simulink model "h2omnix"  (R2023a)
settings: Solver=ode4  StartTime=0.0  StopTime=inf  RelTol=1e-3
undefined symbols (not defined in the file or in its folder): K_av, Kd_pose, Ki_vel, Kp_pose, Kp_vel
libraries: ros2lib x4, MarineRoboticsLib_2 x3, robotcorelib x1
settings Model: Creator=dnad  LastModifiedBy=Enio
settings OptimizationCC: ReuseModelBlockBuffer=off

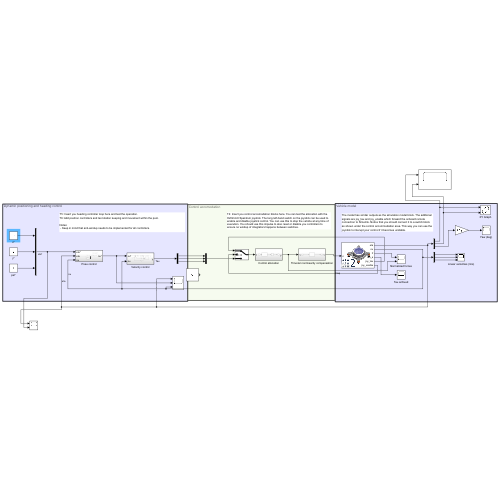
[thumbnail: Simulink's stored preview of the top-level diagram]
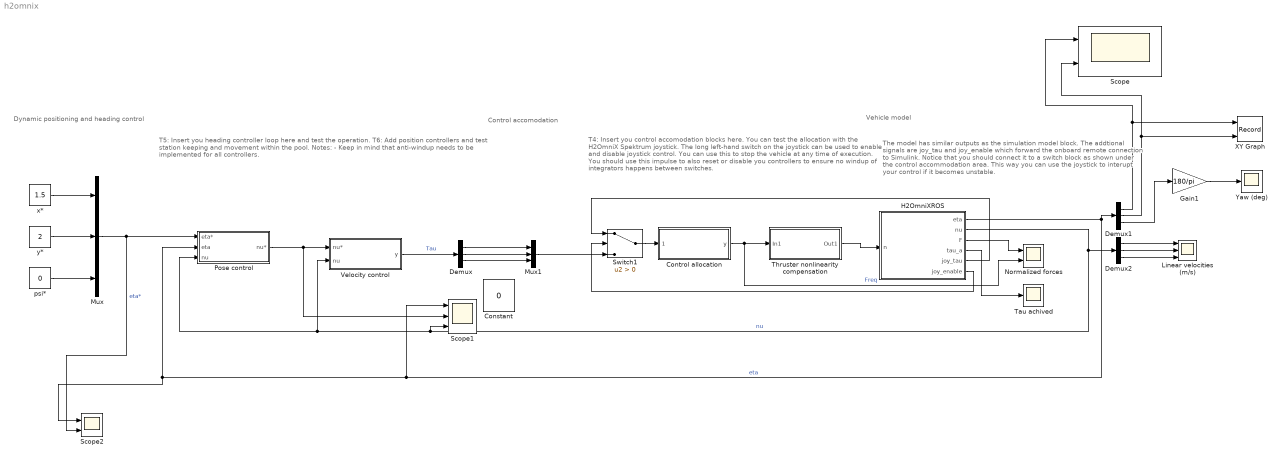
== system h2omnix ==
  note: Control accomodation
  note: T4: Insert you control accomodation blocks here. You can test the allocation with the
      | H2OmniX Spektrum joystick. The long left-hand switch on the joystick can be used to enable and disable joystick control. You can use this to stop the vehicle at any time of execution. You should use this impulse to also reset or disable you controllers to ensure no windup of integrators happens between switches.
  note: Dynamic positioning and heading control
  note: Vehicle model
  note: T5: Insert you heading controller loop here and test the operation.
      | T6: Add position controllers and test station keeping and movement within the pool.
      |
      | Notes:
      |  - Keep in mind that anti-windup needs to be implemented for all controllers.
  note: The model has similar outputs as the simulation model block. The addtional
      | signals are joy_tau and joy_enable which forward the onboard remote
      | connection to Simulink. Notice that you should connect it to a switch block
      | as shown under the control accommodation area. This way you can use the
      | joystick to interupt your control if it becomes unstable.
  Constant : Constant  Value=0
  Control allocation : Subsystem
  Demux : Demux  Outputs=3
  Demux1 : Demux  Outputs=3
  Demux2 : Demux  Outputs=3
  Gain1 : Gain  Gain=180/pi
  H2OmniXROS : Subsystem  AncestorBlock=MarineRoboticsLib_2/H2OmniXROS  mask{vehicle_name=vis, max_pwm=1, pwm_topic=/vis/pwm_out, joy_topic=/vis/joy, odometry_topic=/vis/odometry/filtered}
      mask prompts: vehicle_name "Vehicle name"; max_pwm "Maximum allowed PWM"; pwm_topic "Command"; joy_topic "Joystick"; odometry_topic "Odometry"
      mask init:
      | set_param(gcb, 'pwm_topic',strcat('/', vehicle_name, '/pwm_out'));
      |     set_param(gcb, 'odometry_topic', strcat('/', vehicle_name, '/odometry/filtered'));
      |     set_param(gcb, 'joy_topic', strcat('/', vehicle_name, '/joy'));
      settings: LibrarySourceBlock=MarineRoboticsLib_2/H2OmniXROS
      mask TypeOptions pwm_topic: PublishToROS/topic
      mask TypeOptions joy_topic: Subscribe2/topic
      mask TypeOptions odometry_topic: Subscribe1/topic
      mask DialogControl G1 Prompt: Topics
      mask Display: image('$imagefile'); % Use "Edit Image" on toolstrip to change.
  Linear velocities (m/s) : Scope  NumInputPorts=3
  Mux : Mux  Inputs=3
  Mux1 : Mux  Inputs=3
  Normalized forces : Scope  NumInputPorts=2
  Pose control : Subsystem
  Scope : Scope  NumInputPorts=2
  Scope1 : Scope  NumInputPorts=3
  Scope2 : Scope  NumInputPorts=2
  Switch1 : Switch  Criteria=u2 > Threshold  SaturateOnIntegerOverflow=off  InputSameDT=off
  Tau achived : Scope
  Thruster nonlinearity compensation : Subsystem
  Velocity control : Subsystem
  XY Graph : Record  FileSettingsInternal="{\"entries\":[{\"content\":{\"excelSettings\":{\"content\":{},\"type\":\"Streamout.ExcelSettings\"}},\"type\":\"Streamout.FileSettingStorage\",\"uuid\":\"\"}],\"packageUris\":[\"http:\\/\\/schema.mathworks.com\\/mf0\\/streamout_blocks\\/R2020a\"],\"version\":\"1.0\"}"  Layout=[1 1]  SignalsInternal="{\"entries\":[{\"content\":{\"signals\":[{\"content\":{\"blockPath\":[],\"dimensions\":[1,1],\"domain\":\"\",\"lineColor\":\"#a2142f\",\"plots\":[1],\"port\":1,\"sid\":[\"\"],\"signalID\":29427,\"signalName\":\"Demux1:1\"},\"type\":\"RecordBlkView.Signal\",\"uuid\":\"\"},{\"content\":{\"blockPath\":[],\"dimensions\":[1,1],\"domain\":\"\",\"lineColor\":\"#139fff\",\"plots\":[1],\"port\":2,\"sid\":[\"\"],\"signalID\":29431,\"signalName\":\"Demux1:2\"},\"type\":\"RecordBlkView.Signal\",\"uuid\":\"\"}]},\"type\":\"RecordBlkView.InputSignals\",\"uuid\":\"\"}],\"packageUris\":[\"http:\\/\\/schema.mathworks.com\\/mf0\\/streamout_blocks\\/R2020a\"],\"version\":\"1.0\"}"  VisualizationBindings="{\"xyplotplugin\":{\"info\":[{\"series\":[{\"bindingParametersList\":[{\"parameter\":\"X-Axis\",\"signalID\":29427,\"signalName\":\"Demux1:1\"},{\"parameter\":\"Y-Axis\",\"signalID\":29431,\"signalName\":\"Demux1:2\"}],\"seriesID\":31628}],\"subplotID\":1}]}}"  CompatibilityTag=XY
  Yaw (deg) : Scope
  psi* : Constant  Value=0
  x* : Constant  Value=1.5
  y* : Constant  Value=2
  wires:
  Demux2/1 -> Linear velocities (m/s)/1
  H2OmniXROS/4(tau_a) -> Tau achived/1
  y*/1 -> Mux/2
  Thruster nonlinearity compensation/1(Out1) -> H2OmniXROS/1(n)
  H2OmniXROS/1(eta) -> Scope1/1, Pose control/2(eta), Scope2/1, Demux1/1  "eta"
  Control allocation/1(y) -> Thruster nonlinearity compensation/1(In1), Normalized forces/2  "Freq"
  psi*/1 -> Mux/3
  H2OmniXROS/3(F) -> Normalized forces/1
  Demux1/2 -> XY Graph/2, Scope/2
  H2OmniXROS/2(nu) -> Scope1/3, Pose control/3(nu), Velocity control/2(nu), Demux2/1  "nu"
  Demux1/1 -> XY Graph/1, Scope/1
  Gain1/1 -> Yaw (deg)/1
  Demux1/3 -> Gain1/1
  Demux2/2 -> Linear velocities (m/s)/2
  x*/1 -> Mux/1
  Demux2/3 -> Linear velocities (m/s)/3
  Switch1/1 -> Control allocation/1(1)
  H2OmniXROS/6(joy_enable) -> Switch1/2
  H2OmniXROS/5(joy_tau) -> Switch1/1
  Velocity control/1(y) -> Demux/1  "Tau"
  Mux1/1 -> Switch1/3
  Mux/1 -> Scope2/2, Pose control/1(eta*)  "eta*"
  Pose control/1(nu*) -> Scope1/2, Velocity control/1(nu*)
  Demux/1 -> Mux1/1
  Demux/2 -> Mux1/2
  Demux/3 -> Mux1/3

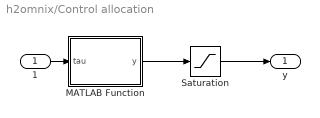
== system h2omnix/Control allocation ==
  1 : Inport
  MATLAB Function : MATLAB Function  TreatAsAtomicUnit=on
  Saturation : Saturate  UpperLimit=1  LowerLimit=-1
  y : Outport
  wires:
  1/1 -> MATLAB Function/1(tau)
  MATLAB Function/1(y) -> Saturation/1
  Saturation/1 -> y/1

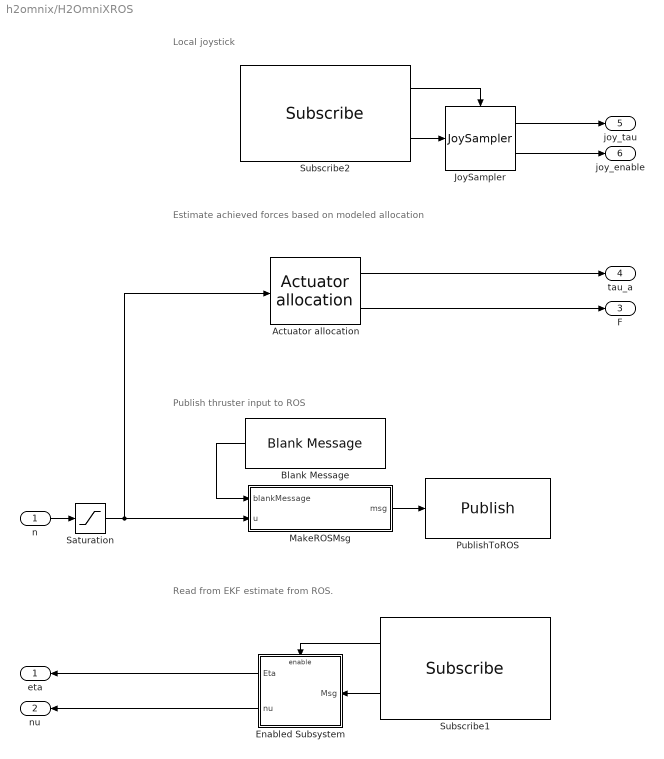
== system h2omnix/H2OmniXROS ==
  note: Local joystick
  note: Read from EKF estimate from ROS.
  note: Publish thruster input to ROS
  note: Estimate achieved forces based on modeled allocation
  n : Inport
  Actuator allocation : MarineRoboticsLib_2/Actuator allocation  Tm=0  B="[0.25, 0.25, -0.25, -0.25; -0.25,  0.25, -0.25,  0.25; -0.25, 0.25, 0.25, -0.25]"  Keff=[1,1,1,1]
  Blank Message : ros2lib/Blank Message  messageClass=Message  entityType=std_msgs/Float32MultiArray  messageType=std_msgs/Float32MultiArray  SampleTime=0.05
  Enabled Subsystem : Subsystem  TreatAsAtomicUnit=on
  JoySampler : MarineRoboticsLib_2/JoyOverROS/JoySampler  SystemSampleTime=-1  VariantActivationTime=update diagram  Latency=0  AutoFrameSizeCalculation=off
  MakeROSMsg : MATLAB Function  TreatAsAtomicUnit=on  SystemSampleTime=0.05
  PublishToROS : ros2lib/Publish  topicSource=Select from ROS network  topic=/vis/pwm_out  messageType=std_msgs/Float32MultiArray  QOSHistory=Keep last  QOSDepth=1  QOSReliability=Reliable  QOSDurability=Volatile
  Saturation : Saturate  UpperLimit=max_pwm  LowerLimit=-max_pwm
  Subscribe1 : ros2lib/Subscribe  topicSource=Specify your own  topic=/vis/odometry/filtered  messageType=nav_msgs/Odometry  sampleTime=0.05  QOSHistory=Keep last  QOSDepth=1  QOSReliability=Reliable  QOSDurability=Volatile
  Subscribe2 : ros2lib/Subscribe  topicSource=Specify your own  topic=/vis/joy  messageType=sensor_msgs/Joy  sampleTime=0.05  QOSHistory=Keep last  QOSDepth=1  QOSReliability=Reliable  QOSDurability=Volatile
  eta : Outport
  nu : Outport  Port=2
  F : Outport  Port=3
  tau_a : Outport  Port=4
  joy_tau : Outport  Port=5
  joy_enable : Outport  Port=6
  wires:
  Saturation/1 -> Actuator allocation/1, MakeROSMsg/2(u)
  MakeROSMsg/1(msg) -> PublishToROS/1
  Subscribe1/2 -> Enabled Subsystem/1(Msg)
  Subscribe1/1 -> Enabled Subsystem/Enable
  Enabled Subsystem/1(Eta) -> eta/1
  Blank Message/1 -> MakeROSMsg/1(blankMessage)
  n/1 -> Saturation/1
  Enabled Subsystem/2(nu) -> nu/1
  Actuator allocation/2 -> F/1
  Actuator allocation/1 -> tau_a/1
  JoySampler/2 -> joy_enable/1
  Subscribe2/2 -> JoySampler/1
  JoySampler/1 -> joy_tau/1
  Subscribe2/1 -> JoySampler/Enable

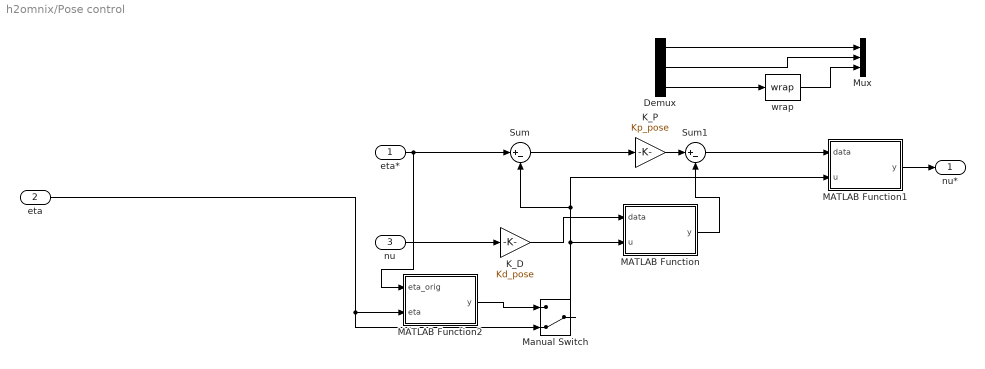
== system h2omnix/Pose control ==
  eta* : Inport
  eta : Inport  Port=2
  nu : Inport  Port=3
  Demux : Demux  Outputs=3
  K_D : Gain  Gain=Kd_pose
  K_P : Gain  Gain=Kp_pose
  MATLAB Function : MATLAB Function  TreatAsAtomicUnit=on
  MATLAB Function1 : MATLAB Function  TreatAsAtomicUnit=on
  MATLAB Function2 : MATLAB Function  TreatAsAtomicUnit=on
  Manual Switch : ManualSwitch  CurrentSetting=0
  Mux : Mux  Inputs=3
  Sum : Sum  Inputs=|+-
  Sum1 : Sum  Inputs=|+-
  wrap : MarineRoboticsLib_2/wrap  SystemSampleTime=-1  VariantActivationTime=update diagram  Latency=0  AutoFrameSizeCalculation=off
      settings: LibrarySourceBlock=|
      | simulink/User-Defined
      | Functions/MATLAB Function
  nu* : Outport
  wires:
  eta*/1 -> MATLAB Function2/1(eta_orig), Sum/1
  nu/1 -> K_D/1
  K_D/1 -> MATLAB Function/1(data)
  MATLAB Function/1(y) -> Sum1/2
  MATLAB Function1/1(y) -> nu*/1
  eta/1 -> Manual Switch/2, MATLAB Function2/2(eta)
  MATLAB Function2/1(y) -> Manual Switch/1
  Manual Switch/1 -> MATLAB Function/2(u), MATLAB Function1/2(u), Sum/2
  Demux/3 -> wrap/1
  wrap/1 -> Mux/3
  Demux/1 -> Mux/1
  Demux/2 -> Mux/2
  Sum1/1 -> MATLAB Function1/1(data)
  K_P/1 -> Sum1/1
  Sum/1 -> K_P/1

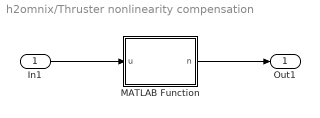
== system h2omnix/Thruster nonlinearity compensation ==
  In1 : Inport
  MATLAB Function : MATLAB Function  TreatAsAtomicUnit=on
  Out1 : Outport
  wires:
  In1/1 -> MATLAB Function/1(u)
  MATLAB Function/1(n) -> Out1/1

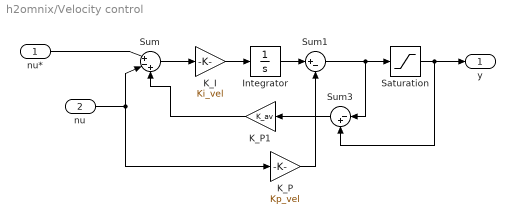
== system h2omnix/Velocity control ==
  nu* : Inport
  nu : Inport  Port=2
  Integrator : Integrator
  K_I : Gain  Gain=Ki_vel
  K_P : Gain  Gain=Kp_vel
  K_P1 : Gain  Gain=K_av
  Saturation : Saturate
  Sum : Sum  Inputs=|+-+
  Sum1 : Sum  Inputs=|+-
  Sum3 : Sum  Inputs=|-+
  y : Outport
  wires:
  nu*/1 -> Sum/1
  nu/1 -> K_P/1, Sum/2
  K_P/1 -> Sum1/2
  Sum1/1 -> Sum3/1, Saturation/1
  Saturation/1 -> y/1, Sum3/2
  Integrator/1 -> Sum1/1
  Sum3/1 -> K_P1/1
  K_I/1 -> Integrator/1
  Sum/1 -> K_I/1
  K_P1/1 -> Sum/3

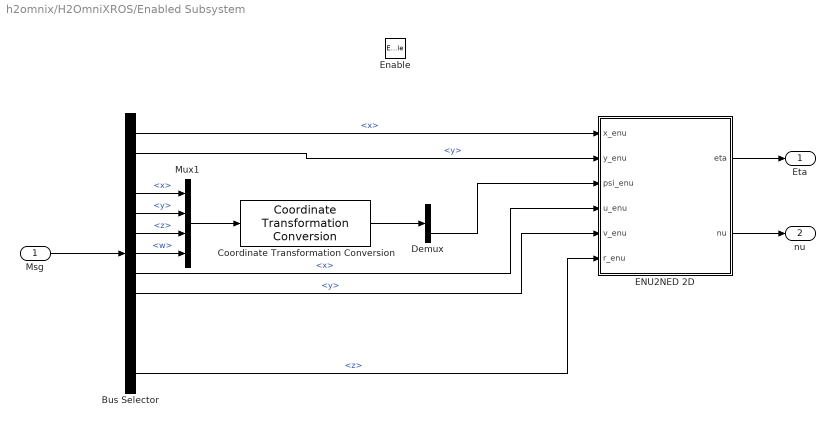
== system h2omnix/H2OmniXROS/Enabled Subsystem ==
  Msg : Inport
  Enable : EnablePort
  Bus Selector : BusSelector  OutputSignals=pose.pose.position.x,pose.pose.position.y,pose.pose.position.z,pose.pose.orientation.x,pose.pose.orientation.y,pose.pose.orientation.z,pose.pose.orientation.w,twist.twist.linear.x,twist.twist.linear.y,twist.twist.linear.z,twist.twist.angular.x,twist.twist.angular.y,twist.twist.angular.z
  Coordinate Transformation Conversion : robotcorelib/Coordinate Transformation Conversion  InputRepresentation=Quaternion  InputEulerSequence=ZYX  ShowTrVecInputPort=on  OutputRepresentation=Euler Angles  OutputEulerSequence=ZYX  ShowTrVecOutputPort=on  SimulateUsing=Interpreted execution
      settings: LibrarySourceBlock=roslib/Utilities/Coordinate Transformation Conversion
  Demux : Demux  Outputs=3
  ENU2NED 2D : MATLAB Function  TreatAsAtomicUnit=on
  Mux1 : Mux
  Eta : Outport
  nu : Outport  Port=2
  wires:
  Msg/1 -> Bus Selector/1
  Bus Selector/4 -> Mux1/1  "<x>"
  Bus Selector/5 -> Mux1/2  "<y>"
  Bus Selector/6 -> Mux1/3  "<z>"
  Bus Selector/7 -> Mux1/4  "<w>"
  Mux1/1 -> Coordinate Transformation Conversion/1
  Bus Selector/2 -> ENU2NED 2D/2(y_enu)  "<y>"
  Bus Selector/1 -> ENU2NED 2D/1(x_enu)  "<x>"
  Coordinate Transformation Conversion/1 -> Demux/1
  Bus Selector/8 -> ENU2NED 2D/4(u_enu)  "<x>"
  Bus Selector/9 -> ENU2NED 2D/5(v_enu)  "<y>"
  Bus Selector/13 -> ENU2NED 2D/6(r_enu)  "<z>"
  ENU2NED 2D/1(eta) -> Eta/1
  ENU2NED 2D/2(nu) -> nu/1
  Demux/3 -> ENU2NED 2D/3(psi_enu)

== matlab function h2omnix/Thruster nonlinearity compensation/MATLAB Function ==
  data: u input; n output
function n = fcn(u)

for i = 1:length(u)
    if u(i) > 1
        u(i) = 1;
    end
end

p1 = 0.5869;
p2 = -0.9109;
p3 = -0.3809;
p4 = 1.6743;
p5 = -0.0089;

n = p1*u.^4 + p2*u.^3 + p3*u.^2 + p4*u + p5;

== matlab function h2omnix/Control allocation/MATLAB Function ==
  data: tau input; y output
function y = fcn(tau)

B = [0.25, 0.25, -0.25, -0.25; -0.25,  0.25, -0.25,  0.25; -0.25, 0.25, 0.25, -0.25];

y = pinv(B)*tau;

end

== matlab function h2omnix/Pose control/MATLAB Function1 ==
  data: data input; u input; y output
function y = fcn(data, u)
%data = [u, v, d_psi]
%u = [x, y, psi]
psi = u(3);
R = [cos(psi), -sin(psi), 0;
     sin(psi), cos(psi),  0;
        0,         0,     1];
y = R'*data;

== matlab function h2omnix/Pose control/MATLAB Function ==
  data: data input; u input; y output
function y = fcn(data, u)
%data = [u, v, d_psi]
%u = [x, y, psi]
psi = u(3);
R = [cos(psi), -sin(psi), 0;
     sin(psi), cos(psi),  0;
        0,         0,     1];
y = R*data;

== matlab function h2omnix/H2OmniXROS/Enabled Subsystem/ENU2NED 2D ==
  data: x_enu input; eta output; y_enu input; psi_enu input; u_enu input; v_enu input; r_enu input; nu output
function [eta, nu] = enu2ned2d(x_enu,y_enu,psi_enu,u_enu,v_enu,r_enu)
% Just do coordinate swap
psi_ned = pi/2-psi_enu;

psi_ned = mod(psi_ned, 2*pi);

if psi_ned > pi
   psi_ned = -2*pi + psi_ned;
elseif psi_ned <= -pi 
   psi_ned = 2*pi + psi_ned;
end


eta = [y_enu; x_enu; psi_ned];
nu = [u_enu; -v_enu; -r_enu;];

== matlab function h2omnix/Pose control/MATLAB Function2 ==
  data: eta_orig input; eta input size=3; y output
function y   = fcn(eta_orig , eta )

if abs(eta_orig(1) - eta(1)) < 0.2 | abs(eta_orig(2) - eta(2)) < 0.2 
    y = eta_orig;
else
    y = eta;
end
end

== matlab function h2omnix/H2OmniXROS/MakeROSMsg ==
  data: blankMessage input; u input; msg output Bus: SL_Bus_std_msgs_Float32MultiArray
function msg  = assign_bus(blankMessage,u)

% blank message input
msg = blankMessage;

% assign pwm values into data field
msg.data(1:numel(u)) = reshape(u,[],1);

% all other fields must be assigned to complete the message
msg.data_SL_Info.CurrentLength = uint32(numel(u));
msg.layout.dim(1).size = uint32(size(u,1));
msg.layout.dim(2).size = uint32(size(u,2));
msg.layout.dim(1).stride = uint32(numel(u));
msg.layout.dim(2).stride = uint32(prod(size(u,2)));
